simulink model "InverterFOCModel"  (R2020b)
settings: Solver=VariableStepAuto  StartTime=0.0  StopTime=10.0  RelTol=1e-3
libraries: nesl_utility x16, ee_lib x15, fl_lib x14, eeTransforms x2, mcbcontrolslib x2, eePmsmCurrentController x1, powerlib_meascontrol x1, eeVelocityController x1
settings Model: Creator=trgre  LastModifiedBy=trgre

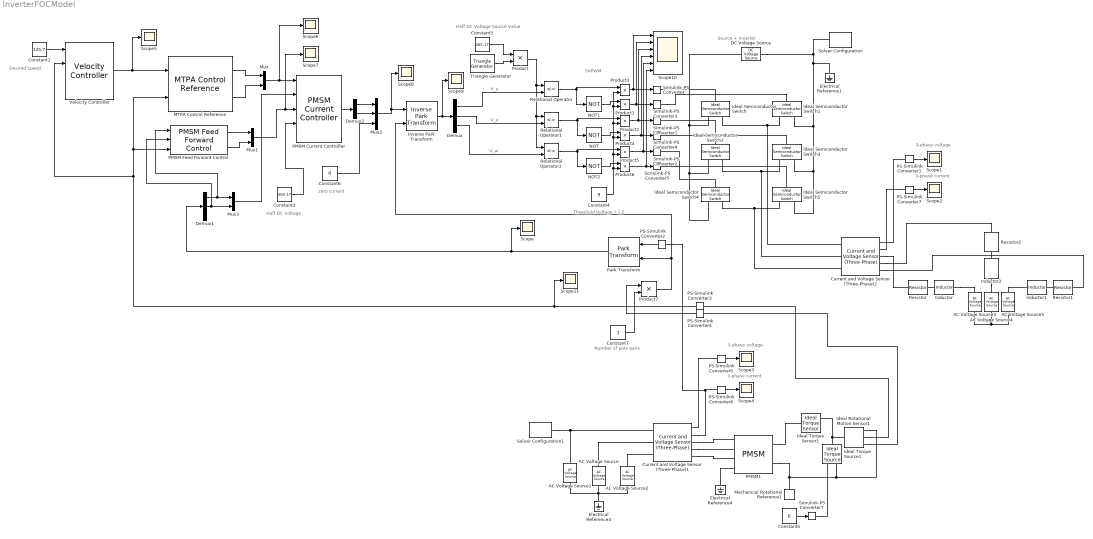
== system InverterFOCModel ==
  note: Number of pole pairs
  note: Desired Speed
  note: Half DC Voltage
  note: zero current
  note: Threshold Voltage * 1.5
  note: Half DC Voltage Source Value
  note: Source + Inverter
  note: SVPWM
  note: V_w
  note: V_v
  note: V_u
  note: 3-phase voltage
  note: 3-phase current
  note: 3-phase voltage
  note: 3-phase current
  AC Voltage Source : fl_lib/Electrical/Electrical Sources/AC Voltage Source  amp=265.17 V  shift=-120 deg  frequency=60 Hz  omega=0 rad/s
  AC Voltage Source1 : fl_lib/Electrical/Electrical Sources/AC Voltage Source  amp=265.17 V  shift=0 deg  frequency=60 Hz  omega=0 rad/s
  AC Voltage Source2 : fl_lib/Electrical/Electrical Sources/AC Voltage Source  amp=265.17 V  shift=120 deg  frequency=60 Hz  omega=0 rad/s
  AC Voltage Source3 : fl_lib/Electrical/Electrical Sources/AC Voltage Source  amp=256 V  shift=0 deg  frequency=60 Hz  omega=0 rad/s
  AC Voltage Source4 : fl_lib/Electrical/Electrical Sources/AC Voltage Source  amp=256 V  shift=-120 deg  frequency=60 Hz  omega=0 rad/s
  AC Voltage Source5 : fl_lib/Electrical/Electrical Sources/AC Voltage Source  amp=256 V  shift=120 deg  frequency=60 Hz  omega=0 rad/s
  Constant1 : Constant  Value=125.7
  Constant2 : Constant  Value=265.17
  Constant3 : Constant  Value=265.17
  Constant4 : Constant  Value=9
  Constant5 : Constant  Value=0
  Constant6 : Constant  Value=0
  Constant7 : Constant  Value=3
  Current and Voltage Sensor (Three-Phase)1 : ee_lib/Sensors & Transducers/Current and Voltage Sensor (Three-Phase)  vMeasurementType=ee.enum.vmeasurement.lg  outputUnit=ee.enum.unit.si  SRated=100e6 V*A  VRated=24e3 V  I_specify=off  I_priority=None  I=[ 0 0 0 ] A  I_nominal_specify=off  I_nominal_unit=A  I_nominal_value=1  V_specify=off  V_priority=None  V=[ 0 0 0 ] V  V_nominal_specify=off  V_nominal_unit=V  V_nominal_value=1
      settings: SourceProductBaseCode=PS  InternalSimscapePortConfiguration="{\"Bottom\":[],\"Left\":[{\"id\":\"a1\",\"label\":\"a1\",\"type\":\"foundation.electrical.electrical\"},{\"id\":\"b1\",\"label\":\"b1\",\"type\":\"foundation.electrical.electrical\"},{\"id\":\"c1\",\"label\":\"c1\",\"type\":\"foundation.electrical.electrical\"}],\"Right\":[{\"id\":\"V_output\",\"label\":\"V\",\"type\":\"output\"},{\"id\":\"I_output\",\"label\":\"I\",\"type\":\"output\"},{\"id\":\"a2\",\"label\":\"a2\",\"type\":\"foundation.electrical.electrical\"},{\"id\":\"b2\",\"label\":\"b2\",\"type\":\"foundation.electrical.electrical\"},{\"id\":\"c2\",\"label\":\"c2\",\"type\":\"foundation.electrical.electrical\"}],\"Top\":[]}"
  Current and Voltage Sensor (Three-Phase)2 : ee_lib/Sensors & Transducers/Current and Voltage Sensor (Three-Phase)  vMeasurementType=ee.enum.vmeasurement.lg  outputUnit=ee.enum.unit.si  SRated=100e6 V*A  VRated=24e3 V  I_specify=off  I_priority=None  I=[ 0 0 0 ] A  I_nominal_specify=off  I_nominal_unit=A  I_nominal_value=1  V_specify=off  V_priority=None  V=[ 0 0 0 ] V  V_nominal_specify=off  V_nominal_unit=V  V_nominal_value=1
      settings: SourceProductBaseCode=PS  InternalSimscapePortConfiguration="{\"Bottom\":[],\"Left\":[{\"id\":\"a1\",\"label\":\"a1\",\"type\":\"foundation.electrical.electrical\"},{\"id\":\"b1\",\"label\":\"b1\",\"type\":\"foundation.electrical.electrical\"},{\"id\":\"c1\",\"label\":\"c1\",\"type\":\"foundation.electrical.electrical\"}],\"Right\":[{\"id\":\"V_output\",\"label\":\"V\",\"type\":\"output\"},{\"id\":\"I_output\",\"label\":\"I\",\"type\":\"output\"},{\"id\":\"a2\",\"label\":\"a2\",\"type\":\"foundation.electrical.electrical\"},{\"id\":\"b2\",\"label\":\"b2\",\"type\":\"foundation.electrical.electrical\"},{\"id\":\"c2\",\"label\":\"c2\",\"type\":\"foundation.electrical.electrical\"}],\"Top\":[]}"
  DC Voltage Source : fl_lib/Electrical/Electrical Sources/DC Voltage Source  v0=530.35 V
  Demux : Demux  Outputs=3
  Demux1 : Demux  Outputs=3
  Demux2 : Demux  Outputs=2
  Electrical Reference1 : fl_lib/Electrical/Electrical Elements/Electrical Reference
  Electrical Reference3 : fl_lib/Electrical/Electrical Elements/Electrical Reference
  Electrical Reference4 : fl_lib/Electrical/Electrical Elements/Electrical Reference
  Ideal Rotational Motion Sensor1 : fl_lib/Mechanical/Mechanical Sensors/Ideal Rotational Motion Sensor  wrap_angle=simscape.enum.onoff.off  offset=0 rad
  Ideal Semiconductor Switch{,1..5} (6 alike) : ee_lib/Semiconductors & Converters/Ideal Semiconductor Switch  Ron=0.001 Ohm  Goff=1e-6 1/Ohm  Vth=6 V  diode_param=2  diode_Vf=0.8 V  diode_Ron=0.001 Ohm  diode_Goff=1e-5 1/Ohm  diode_C=50e-9 F  diode_iRM=-235 A  diode_iF=300 A  diode_idot=-50 A/us  diode_trr_param=1  diode_trr_factor=3  diode_trr=15 us  diode_Qrr=1500 s*uA
      settings: SourceProductBaseCode=PS
  Ideal Torque Sensor1 : fl_lib/Mechanical/Mechanical Sensors/Ideal Torque Sensor
  Ideal Torque Source1 : fl_lib/Mechanical/Mechanical Sources/Ideal Torque Source
  Inductor : ee_lib/Passive/Inductor  l=0.00137 H  L_tol=0  enable_L_tol=0  tol_distribution=1  nSigma=4  r=0 Ohm  g=1e-9 1/Ohm  enable_operating_limits=0  operating_limit_action=2  max_working_current=1 A  power_rating=1 W  enable_faults=0  fault_action=1  lambdaPercent=50  k_faulted=0.9999  turnsShort=0  openCct=0  groundShort=0  groundShortG=0 1/Ohm  tau_fault=1e-3 s  enable_temporal_fault=0  t_fault=1 s  enable_behavioral_fault=0  max_permissible_voltage=100 V  n_fail_on_voltage=1  max_permissible_current=1 A  t_fail_on_current=1 s  i_L_specify=off  i_L_priority=High  i_L=0 A  i_L_nominal_specify=off  i_L_nominal_unit=A  i_L_nominal_value=1
  Inductor1 : ee_lib/Passive/Inductor  l=0.00137 H  L_tol=0  enable_L_tol=0  tol_distribution=1  nSigma=4  r=0 Ohm  g=1e-9 1/Ohm  enable_operating_limits=0  operating_limit_action=2  max_working_current=1 A  power_rating=1 W  enable_faults=0  fault_action=1  lambdaPercent=50  k_faulted=0.9999  turnsShort=0  openCct=0  groundShort=0  groundShortG=0 1/Ohm  tau_fault=1e-3 s  enable_temporal_fault=0  t_fault=1 s  enable_behavioral_fault=0  max_permissible_voltage=100 V  n_fail_on_voltage=1  max_permissible_current=1 A  t_fail_on_current=1 s  i_L_specify=off  i_L_priority=High  i_L=0 A  i_L_nominal_specify=off  i_L_nominal_unit=A  i_L_nominal_value=1
  Inductor2 : ee_lib/Passive/Inductor  l=0.00137 H  L_tol=0  enable_L_tol=0  tol_distribution=1  nSigma=4  r=0 Ohm  g=1e-9 1/Ohm  enable_operating_limits=0  operating_limit_action=2  max_working_current=1 A  power_rating=1 W  enable_faults=0  fault_action=1  lambdaPercent=50  k_faulted=0.9999  turnsShort=0  openCct=0  groundShort=0  groundShortG=0 1/Ohm  tau_fault=1e-3 s  enable_temporal_fault=0  t_fault=1 s  enable_behavioral_fault=0  max_permissible_voltage=100 V  n_fail_on_voltage=1  max_permissible_current=1 A  t_fail_on_current=1 s  i_L_specify=off  i_L_priority=High  i_L=0 A  i_L_nominal_specify=off  i_L_nominal_unit=A  i_L_nominal_value=1
  Inverse Park Transform : eeTransforms/Inverse Park Transform  AxisAlignment=Q-axis  PowerInvariant=off
  MTPA Control Reference : mcbcontrolslib/MTPA Control Reference  LabelModeActiveChoice=Surface PMSM  VariantSelect=Surface PMSM  polePairs=3  Rs=0.36  Ld=0.0024  Lq=0.4e-3  FluxPM=0.048  I_sat=7.1  V_dc=24  Units=SI Units  N_base=1200  I_base=19.3  T_base=1  N_base_disp=3182
      settings: SourceProductBaseCode=MT
  Mechanical Rotational Reference1 : fl_lib/Mechanical/Rotational Elements/Mechanical Rotational Reference
  Mux : Mux  Inputs=2
  Mux1 : Mux  Inputs=2
  Mux2 : Mux  Inputs=3
  Mux3 : Mux  Inputs=2
  NOT : Logic  Operator=NOT  IconShape=distinctive  AllPortsSameDT=off  OutDataTypeStr=boolean
  NOT1 : Logic  Operator=NOT  IconShape=distinctive  AllPortsSameDT=off  OutDataTypeStr=boolean
  NOT2 : Logic  Operator=NOT  IconShape=distinctive  AllPortsSameDT=off  OutDataTypeStr=boolean
  PMSM Current Controller : eePmsmCurrentController/PMSM Current Controller  Kp_id=1  Ki_id=100  Kaw_id=1  Kp_iq=1  Ki_iq=100  Kaw_iq=1  Ts=-1  Tsd=0.001  AxisPrio=Q-axis  ActZC=off  ActFF=on
      settings: SourceProductBaseCode=PS
  PMSM Feed Forward Control : mcbcontrolslib/PMSM Feed Forward Control  polePairs=4  Ld=0.2e-3  Lq=0.2e-3  FluxPM=6.4e-3  V_dc=24/sqrt(3)  Units=Per-Unit (PU)  V_base=24/sqrt(3)  I_base=19.3  N_base=4107
      settings: SourceProductBaseCode=MT
  PMSM1 : ee_lib/Electromechanical/Permanent Magnet/PMSM  winding_type=ee.enum.statorconnection.wye  machine_param=ee.enum.pmsm.parameterization.constant  nPolePairs=3  pmflux_param=ee.enum.pmflux.fluxlinkage  pm_flux_linkage=0.48 Wb  torque_constant=0.76 N*m/A  back_emf_constant=0.18 V/(rad/s)  stator_param=ee.enum.statorparam.LdLqL0  Ld=0.00137 H  Lq=0.00137 H  idVec=[-200, 0, 200] A  iqVec=[-200, 0, 200] A  LdMatrix=0.0002 * ones(3, 3) H  LqMatrix=0.0002 * ones(3, 3) H  PmMatrix=0.1 * ones(3, 3) Wb  ktMatrix=0.18 * ones(3, 3) N*m/A  keMatrix=0.18 * ones(3, 3) V/(rad/s)  L0=0.00137 H  Ls=0.0002 H  Lm=-0.00002 H  Ms=0.00002 H  Rs=0.001 Ohm  zero_sequence=ee.enum.park.zerosequence.include  J=0.01 kg*m^2  lam=0.5 N*m/(rad/s)  axes_param=ee.enum.rotorangle.daxis  i_d_specify=off  i_d_priority=None  i_d=1 A  i_d_nominal_specify=off  i_d_nominal_unit=A  i_d_nominal_value=1  i_q_specify=off  i_q_priority=None  i_q=1 A  i_q_nominal_specify=off  i_q_nominal_unit=A  i_q_nominal_value=1  torque_specify=off  torque_priority=None  torque=0 N*m  torque_nominal_specify=off  torque_nominal_unit=N*m  torque_nominal_value=1  angular_velocity_specify=on  angular_velocity_priority=High  angular_velocity=1200 rpm  angular_velocity_nominal_specify=off  angular_velocity_nominal_unit=rpm  angular_velocity_nominal_value=1  angular_position_specify=off  angular_position_priority=High  angular_position=0 deg  angular_position_nominal_specify=off  angular_position_nominal_unit=deg  angular_position_nominal_value=1  loss_param=ee.enum.ironloss.none  losses_oc=[0, 0, 0] W  losses_sc=[0, 0, 0] W  f_losses=60 Hz  Isc_losses=95 A  Tmeas=298.15 K  alpha=3.93e-3 1/K  alpha_flux=-0.001 1/K  stator_thermal_mass=100 J/K  rotor_thermal_mass=200 J/K  Rm_percent_rotor=90  Rd_percent_rotor=30  temperatureA_specify=off  temperatureA_priority=High  temperatureA=25 degC  temperatureA_nominal_specify=off  temperatureA_nominal_unit=degC  temperatureA_nominal_value=1  temperatureB_specify=off  temperatureB_priority=High  temperatureB=25 degC  temperatureB_nominal_specify=off  temperatureB_nominal_unit=degC  temperatureB_nominal_value=1  temperatureC_specify=off  temperatureC_priority=High  temperatureC=25 degC  temperatureC_nominal_specify=off  temperatureC_nominal_unit=degC  temperatureC_nominal_value=1  temperatureR_specify=off  temperatureR_priority=High  temperatureR=25 degC  temperatureR_nominal_specify=off  temperatureR_nominal_unit=degC  temperatureR_nominal_value=1
      settings: InternalSimscapePortConfiguration="{\"Bottom\":[],\"Left\":[{\"id\":\"a\",\"label\":\"a\",\"type\":\"foundation.electrical.electrical\"},{\"id\":\"b\",\"label\":\"b\",\"type\":\"foundation.electrical.electrical\"},{\"id\":\"c\",\"label\":\"c\",\"type\":\"foundation.electrical.electrical\"},{\"id\":\"n\",\"label\":\"n\",\"type\":\"foundation.electrical.electrical\"}],\"Right\":[{\"id\":\"R\",\"label\":\"R\",\"type\":\"foundation.mechanical.rotational.rotational\"},{\"id\":\"C\",\"label\":\"C\",\"type\":\"foundation.mechanical.rotational.rotational\"}],\"Top\":[]}"
  PS-Simulink Converter{1..7} (7 alike) : nesl_utility/PS-Simulink Converter  PhysicalDomain=network_engine_domain  SubClassName=ps_output  LeftPortType=input  RightPortType=output  PseudoPeriodic=off  Frequencies=[]  Unit=inherit  AffineConversion=off
  Park Transform : eeTransforms/Park Transform  AxisAlignment=Q-axis  PowerInvariant=off
  Product{,1..7} (8 alike) : Product
  Relational Operator : RelationalOperator  Operator=<=  OutDataTypeStr=boolean  RndMeth=Simplest
  Relational Operator1 : RelationalOperator  Operator=<=  OutDataTypeStr=boolean  RndMeth=Simplest
  Relational Operator2 : RelationalOperator  Operator=<=  OutDataTypeStr=boolean  RndMeth=Simplest
  Resistor : ee_lib/Passive/Resistor  R=0.001 Ohm  R_tol=5  enable_R_tol=0  tol_distribution=1  nSigma=4  enable_operating_limits=0  operating_limit_action=2  max_working_voltage=100 V  power_rating=1 W  enable_faults=0  fault_action=1  R_faulted=inf Ohm  enable_temporal_fault=0  t_fault=1 s  enable_behavioral_fault=0  max_permissible_current=1 A  t_fail_on_current=1 s  noise_mode=0  sample_time=1e-3 s  repeatability=1  auto_seed=2158918356  user_seed=0  Tdevice=25 degC  alpha=3.93e-3 1/K  Tmeas=25 degC  thermal_mass=100 J/K  power_derating_T1=70 degC  power_derating_T2=155 degC  operating_temperature_range_vec=[-50, 150] degC  temperature_specify=off  temperature_priority=High  temperature=298.15 K  temperature_nominal_specify=off  temperature_nominal_unit=K  temperature_nominal_value=1
  Resistor1 : ee_lib/Passive/Resistor  R=0.001 Ohm  R_tol=5  enable_R_tol=0  tol_distribution=1  nSigma=4  enable_operating_limits=0  operating_limit_action=2  max_working_voltage=100 V  power_rating=1 W  enable_faults=0  fault_action=1  R_faulted=inf Ohm  enable_temporal_fault=0  t_fault=1 s  enable_behavioral_fault=0  max_permissible_current=1 A  t_fail_on_current=1 s  noise_mode=0  sample_time=1e-3 s  repeatability=1  auto_seed=3828569039  user_seed=0  Tdevice=25 degC  alpha=3.93e-3 1/K  Tmeas=25 degC  thermal_mass=100 J/K  power_derating_T1=70 degC  power_derating_T2=155 degC  operating_temperature_range_vec=[-50, 150] degC  temperature_specify=off  temperature_priority=High  temperature=298.15 K  temperature_nominal_specify=off  temperature_nominal_unit=K  temperature_nominal_value=1
  Resistor2 : ee_lib/Passive/Resistor  R=0.001 Ohm  R_tol=5  enable_R_tol=0  tol_distribution=1  nSigma=4  enable_operating_limits=0  operating_limit_action=2  max_working_voltage=100 V  power_rating=1 W  enable_faults=0  fault_action=1  R_faulted=inf Ohm  enable_temporal_fault=0  t_fault=1 s  enable_behavioral_fault=0  max_permissible_current=1 A  t_fail_on_current=1 s  noise_mode=0  sample_time=1e-3 s  repeatability=1  auto_seed=3120255443  user_seed=0  Tdevice=25 degC  alpha=3.93e-3 1/K  Tmeas=25 degC  thermal_mass=100 J/K  power_derating_T1=70 degC  power_derating_T2=155 degC  operating_temperature_range_vec=[-50, 150] degC  temperature_specify=off  temperature_priority=High  temperature=298.15 K  temperature_nominal_specify=off  temperature_nominal_unit=K  temperature_nominal_value=1
  Scope{,1..9,11} (11 alike) : Scope
  Scope10 : Scope  NumInputPorts=6
  Simulink-PS Converter{,1..5,7} (7 alike) : nesl_utility/Simulink-PS Converter  PhysicalDomain=network_engine_domain  SubClassName=ps_input  LeftPortType=input  RightPortType=output  PseudoPeriodic=off  Frequencies=[]  NoiseDistribution=none  NoiseParameters=[]  Unit=1  AffineConversion=off  FilteringAndDerivatives=provide  SimscapeFilterOrder=1  InputFilterTimeConstant=0.001  UdotUserProvided=0
  Solver Configuration : nesl_utility/Solver Configuration  PhysicalDomain=network_engine_domain  SubClassName=solver  LeftPortType=input  RightPortType=generic  Tones=[]  Harmonics=[]  SimulateNoise=off  Profile=off  UseLocalSampling=off  EnableSwitchedLinearOptims=on  FrequencyDomain=off  UseCCode=off  RelTol=0.001  AbsTol=1e-06  MinStep=1e-09  ToWorkspace=off  RevertToSquareIcSolve=off  NumHomotopyIterations=100  PhasorMode=off  PhasorModeNumHarmonics=1  DoDC=off  ResidualTolerance=1e-09  UseLocalSolver=off  LocalSolverChoice=NE_BACKWARD_EULER_ADVANCER  LocalSolverSampleTime=0.001  DoFixedCost=off  MaxNonlinIter=3  MaxModeIter=2  ComputeImpulses=off  ImpulseIterations=2  LinearAlgebra=auto  EquationFormulation=NE_TIME_EF  DelaysMemoryBudget=1024  AutomaticFiltering=on  FilteringTimeConstant=0.001  PartitionStorageMethod=AS_NEEDED  PartitionMemoryBudget=1024  PartitionMethod=ROBUST
  Solver Configuration1 : nesl_utility/Solver Configuration  PhysicalDomain=network_engine_domain  SubClassName=solver  LeftPortType=input  RightPortType=generic  Tones=[]  Harmonics=[]  SimulateNoise=off  Profile=off  UseLocalSampling=off  EnableSwitchedLinearOptims=on  FrequencyDomain=off  UseCCode=off  RelTol=0.001  AbsTol=1e-06  MinStep=1e-09  ToWorkspace=off  RevertToSquareIcSolve=off  NumHomotopyIterations=100  PhasorMode=off  PhasorModeNumHarmonics=1  DoDC=off  ResidualTolerance=1e-09  UseLocalSolver=off  LocalSolverChoice=NE_BACKWARD_EULER_ADVANCER  LocalSolverSampleTime=0.001  DoFixedCost=off  MaxNonlinIter=3  MaxModeIter=2  ComputeImpulses=off  ImpulseIterations=2  LinearAlgebra=auto  EquationFormulation=NE_TIME_EF  DelaysMemoryBudget=1024  AutomaticFiltering=on  FilteringTimeConstant=0.001  PartitionStorageMethod=AS_NEEDED  PartitionMemoryBudget=1024  PartitionMethod=ROBUST
  Triangle Generator : powerlib_meascontrol/Pulse & Signal Generators/Triangle Generator  Freq=10e3  Phase=90  Ts=0
  Velocity Controller : eeVelocityController/Velocity Controller  CtrlType=PI control  Kp_w=1  Ki_w=1  Kv_w=1  Kaw_w=1  Ts=-1  Tsd=0.001  ActZC=off
      settings: SourceProductBaseCode=PS
  wires:
  Demux/1 -> Relational Operator/2
  Relational Operator2/1 -> NOT2/1, Product5/1
  Demux/3 -> Relational Operator2/2
  Relational Operator/1 -> NOT1/1, Product3/1
  Relational Operator1/1 -> NOT/1, Product2/1
  Demux/2 -> Relational Operator1/2
  Inverse Park Transform/1 -> Scope9/1, Demux/1
  PS-Simulink Converter2/1 -> Park Transform/1
  Constant3/1 -> Product/1
  Triangle Generator/1 -> Product/2
  Product/1 -> Relational Operator/1, Relational Operator1/1, Relational Operator2/1
  Product4/1 -> Scope10/4, Simulink-PS Converter4/1
  Product5/1 -> Scope10/5, Simulink-PS Converter2/1
  Product6/1 -> Scope10/6, Simulink-PS Converter5/1
  Product2/1 -> Scope10/3, Simulink-PS Converter1/1
  Product1/1 -> Scope10/2, Simulink-PS Converter3/1
  Product3/1 -> Scope10/1, Simulink-PS Converter/1
  NOT1/1 -> Product1/1
  NOT/1 -> Product4/1
  NOT2/1 -> Product6/1
  Constant4/1 -> Product6/2, Product5/2, Product4/2, Product2/2, Product1/2, Product3/2
  Park Transform/1 -> Scope/1, Demux1/1
  MTPA Control Reference/1 -> Mux/1
  MTPA Control Reference/2 -> Mux/2
  Mux/1 -> Scope6/1, PMSM Current Controller/1
  Velocity Controller/1 -> Scope5/1, MTPA Control Reference/1
  PMSM Feed Forward Control/1 -> Mux1/1
  PMSM Feed Forward Control/2 -> Mux1/2
  Mux1/1 -> Scope7/1, PMSM Current Controller/3
  PS-Simulink Converter3/1 -> Scope11/1, Velocity Controller/2, PMSM Feed Forward Control/3, MTPA Control Reference/2
  PS-Simulink Converter4/1 -> Product7/1
  Constant1/1 -> Velocity Controller/1
  Constant2/1 -> PMSM Current Controller/4
  PS-Simulink Converter6/1 -> Scope4/1
  Constant5/1 -> Simulink-PS Converter7/1
  PS-Simulink Converter5/1 -> Scope3/1
  PMSM Current Controller/1 -> Demux2/1
  Demux2/1 -> Mux2/1
  Demux2/2 -> Mux2/2
  Mux2/1 -> Scope8/1, Inverse Park Transform/1
  Constant6/1 -> Mux2/3
  Demux1/1 -> Mux3/1, PMSM Feed Forward Control/1
  Demux1/2 -> Mux3/2, PMSM Feed Forward Control/2
  Mux3/1 -> PMSM Current Controller/2
  Product7/1 -> Inverse Park Transform/2, Park Transform/2
  Constant7/1 -> Product7/2
  PS-Simulink Converter7/1 -> Scope2/1
  PS-Simulink Converter1/1 -> Scope1/1
  connections:
  Ideal Semiconductor Switch2/RConn1 -- Current and Voltage Sensor (Three-Phase)2/LConn2 -- Ideal Semiconductor Switch3/RConn2
  Ideal Semiconductor Switch4/RConn1 -- Current and Voltage Sensor (Three-Phase)2/LConn3 -- Ideal Semiconductor Switch5/RConn2
  Ideal Semiconductor Switch/RConn2 -- DC Voltage Source/LConn1 -- Ideal Semiconductor Switch2/RConn2 -- Ideal Semiconductor Switch4/RConn2
  Ideal Semiconductor Switch1/RConn2 -- Current and Voltage Sensor (Three-Phase)2/LConn1 -- Ideal Semiconductor Switch/RConn1
  Ideal Semiconductor Switch/LConn1 -- Simulink-PS Converter/RConn1
  Simulink-PS Converter3/RConn1 -- Ideal Semiconductor Switch1/LConn1
  Ideal Semiconductor Switch2/LConn1 -- Simulink-PS Converter1/RConn1
  Ideal Semiconductor Switch3/LConn1 -- Simulink-PS Converter4/RConn1
  Ideal Semiconductor Switch5/LConn1 -- Simulink-PS Converter5/RConn1
  Ideal Semiconductor Switch4/LConn1 -- Simulink-PS Converter2/RConn1
  Ideal Semiconductor Switch5/RConn1 -- Ideal Semiconductor Switch3/RConn1 -- Ideal Semiconductor Switch1/RConn1 -- Electrical Reference1/LConn1 -- DC Voltage Source/RConn1 -- Solver Configuration/RConn1
  Ideal Torque Source1/RConn2 -- Mechanical Rotational Reference1/LConn1 -- PMSM1/RConn2 -- Ideal Rotational Motion Sensor1/RConn1
  Current and Voltage Sensor (Three-Phase)1/RConn2 -- PS-Simulink Converter2/LConn1 -- PS-Simulink Converter6/LConn1
  Ideal Torque Source1/LConn1 -- Ideal Torque Sensor1/RConn1 -- Ideal Rotational Motion Sensor1/LConn1
  Simulink-PS Converter7/RConn1 -- Ideal Torque Source1/RConn1
  Current and Voltage Sensor (Three-Phase)1/RConn5 -- PMSM1/LConn3
  PMSM1/LConn4 -- Electrical Reference4/LConn1
  PMSM1/RConn1 -- Ideal Torque Sensor1/LConn1
  Current and Voltage Sensor (Three-Phase)1/RConn3 -- PMSM1/LConn1
  Current and Voltage Sensor (Three-Phase)1/RConn1 -- PS-Simulink Converter5/LConn1
  Current and Voltage Sensor (Three-Phase)1/RConn4 -- PMSM1/LConn2
  AC Voltage Source1/RConn1 -- Electrical Reference3/LConn1 -- AC Voltage Source/RConn1 -- AC Voltage Source2/RConn1
  AC Voltage Source2/LConn1 -- Current and Voltage Sensor (Three-Phase)1/LConn3
  AC Voltage Source/LConn1 -- Current and Voltage Sensor (Three-Phase)1/LConn2
  AC Voltage Source1/LConn1 -- Current and Voltage Sensor (Three-Phase)1/LConn1 -- Solver Configuration1/RConn1
  Ideal Rotational Motion Sensor1/RConn3 -- PS-Simulink Converter4/LConn1
  Ideal Rotational Motion Sensor1/RConn2 -- PS-Simulink Converter3/LConn1
  AC Voltage Source5/RConn1 -- AC Voltage Source3/RConn1 -- AC Voltage Source4/RConn1
  Resistor2/RConn1 -- Inductor2/LConn1
  Inductor2/RConn1 -- AC Voltage Source4/LConn1
  Inductor1/RConn1 -- AC Voltage Source5/LConn1
  Resistor1/RConn1 -- Inductor1/LConn1
  Inductor/RConn1 -- AC Voltage Source3/LConn1
  Resistor/RConn1 -- Inductor/LConn1
  Current and Voltage Sensor (Three-Phase)2/RConn5 -- Resistor1/LConn1
  Current and Voltage Sensor (Three-Phase)2/RConn4 -- Resistor2/LConn1
  Current and Voltage Sensor (Three-Phase)2/RConn3 -- Resistor/LConn1
  Current and Voltage Sensor (Three-Phase)2/RConn1 -- PS-Simulink Converter1/LConn1
  Current and Voltage Sensor (Three-Phase)2/RConn2 -- PS-Simulink Converter7/LConn1
